simulink model "Manoel_01"  (R2018a)
settings: Solver=VariableStepAuto  StartTime=0.0  StopTime=20  RelTol=1e-3
values from neighbouring files (symbols this model uses):
  A = [-4.5 0; 1 -0.2]    [manoel_outubro2.m]    (also in pre6_teste.m; pre_lab5.m; pre_lab6.m; pre_pedro.m = [-5.5 0; 1 -8.40])
  A1 = ssaux.a    [manoel_outubro2.m]
  atraso = stt    [manoel_outubro2.m]    (also in naao_roda.m = infor.SettlingTime; pre6_teste.m = infor.SettlingTime; pre_lab3.m = infor.SettlingTime; pre_lab3_lab.m = infor.SettlingTime)
  B = [21.6; 0]    [manoel_outubro2.m]    (also in pre6_teste.m; pre_lab5.m = [18; 0]; pre_lab6.m = [b0; 0]; pre_pedro.m = [462; 0])
  B1 = ssaux.b    [manoel_outubro2.m]
  ganho = 0.01027*infor.SettlingMax    [manoel_outubro2.m]    (also in naao_roda.m; pre6_teste.m; pre_lab3.m; pre_lab3_lab.m)
  T0 = round(t0,3)    [naao_roda.m]    (also in pre6_teste.m = 0.063; pre_lab3.m; pre_lab3_2.m = 0.0640576; pre_lab3_lab.m)
undefined symbols (not defined in the file or in its folder): A2, B2
settings Model: Creator=joaovitor  LastModifiedBy=joaovitor

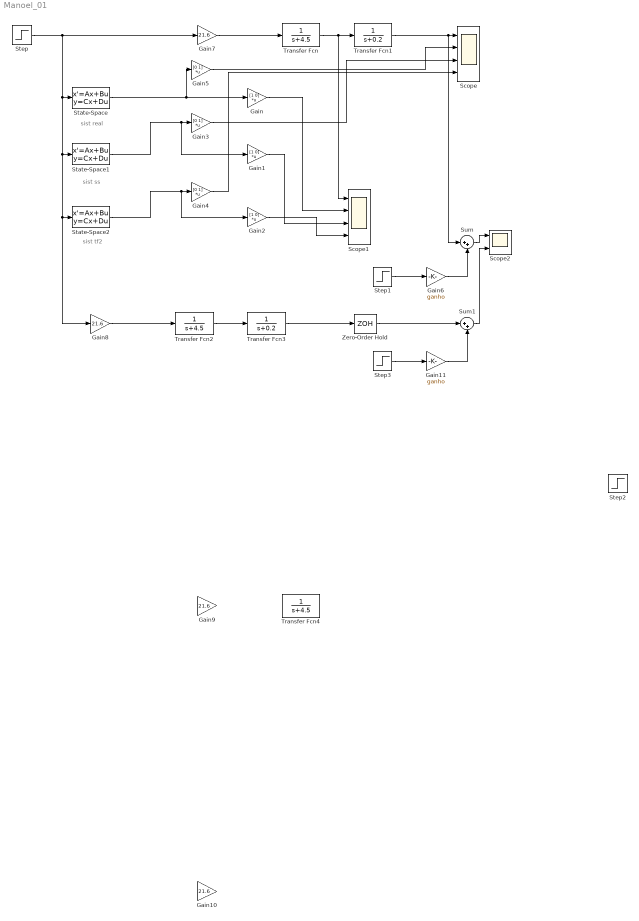
== system Manoel_01 ==
  note: sist tf2
  note: sist ss
  note: sist real
  Gain : Gain  Gain=[1 0]  Multiplication=Matrix(K*u)
  Gain1 : Gain  Gain=[1 0]  Multiplication=Matrix(K*u)
  Gain{7..10} (4 alike) : Gain  Gain=21.6
  Gain11 : Gain  Gain=ganho
  Gain2 : Gain  Gain=[1 0]  Multiplication=Matrix(K*u)
  Gain3 : Gain  Gain=[0 1]  Multiplication=Matrix(K*u)
  Gain4 : Gain  Gain=[0 1]  Multiplication=Matrix(K*u)
  Gain5 : Gain  Gain=[0 1]  Multiplication=Matrix(K*u)
  Gain6 : Gain  Gain=ganho
  Scope : Scope  NumInputPorts=4
  Scope1 : Scope  NumInputPorts=4
  Scope2 : Scope  NumInputPorts=2
  State-Space : StateSpace  A=A  B=B  C=[1 0; 0 1]  D=[0; 0]  InitialCondition=0
  State-Space1 : StateSpace  A=A1  B=B1  C=[1 0; 0 1]  D=[0;0]  InitialCondition=0
  State-Space2 : StateSpace  A=A2  B=B2  C=[1 0; 0 1]  D=[0;0]  InitialCondition=0
  Step : Step  SampleTime=0
  Step1 : Step  Time=1.5*atraso  SampleTime=0
  Step2 : Step  SampleTime=0
  Step3 : Step  Time=1.5*atraso  SampleTime=0
  Sum : Sum  Inputs=|++
  Sum1 : Sum  Inputs=|++
  Transfer Fcn : TransferFcn  Denominator=[1 4.5]
  Transfer Fcn1 : TransferFcn  Denominator=[1 0.2]
  Transfer Fcn2 : TransferFcn  Denominator=[1 4.5]
  Transfer Fcn3 : TransferFcn  Denominator=[1 0.2]
  Transfer Fcn4 : TransferFcn  Denominator=[1 4.5]
  Zero-Order Hold : ZeroOrderHold  SampleTime=T0
  wires:
  Transfer Fcn/1 -> Scope1/1, Transfer Fcn1/1
  Transfer Fcn1/1 -> Sum/1, Scope/1
  Step/1 -> Gain8/1, State-Space2/1, State-Space1/1, State-Space/1, Gain7/1
  State-Space/1 -> Gain5/1, Gain/1
  Gain5/1 -> Scope/2
  Gain3/1 -> Scope/3
  Gain4/1 -> Scope/4
  State-Space1/1 -> Gain1/1, Gain3/1
  State-Space2/1 -> Gain2/1, Gain4/1
  Gain/1 -> Scope1/2
  Gain1/1 -> Scope1/3
  Gain2/1 -> Scope1/4
  Step1/1 -> Gain6/1
  Gain6/1 -> Sum/2
  Sum/1 -> Scope2/1
  Gain7/1 -> Transfer Fcn/1
  Gain11/1 -> Sum1/2
  Step3/1 -> Gain11/1
  Transfer Fcn3/1 -> Zero-Order Hold/1
  Transfer Fcn2/1 -> Transfer Fcn3/1
  Gain8/1 -> Transfer Fcn2/1
  Zero-Order Hold/1 -> Sum1/1
  Sum1/1 -> Scope2/2
